simulink model "impulsestepmodel"  (Simulink 8.3)
settings: Solver=ode23tb  StartTime=0.0  StopTime=100  RelTol=1e-3
settings Model: Creator=NILIMESH GHOSH  LastModifiedBy=NILIMESH GHOSH
settings DataIOCC: SignalLoggingSaveFormat=Dataset
settings DebuggingCC: UnderspecifiedInitializationDetection=Simplified  SolverPrmCheckMsg=none  StateNameClashWarn=none
settings GRTTargetCC: CombineOutputUpdateFcns=on  GRTInterface=off

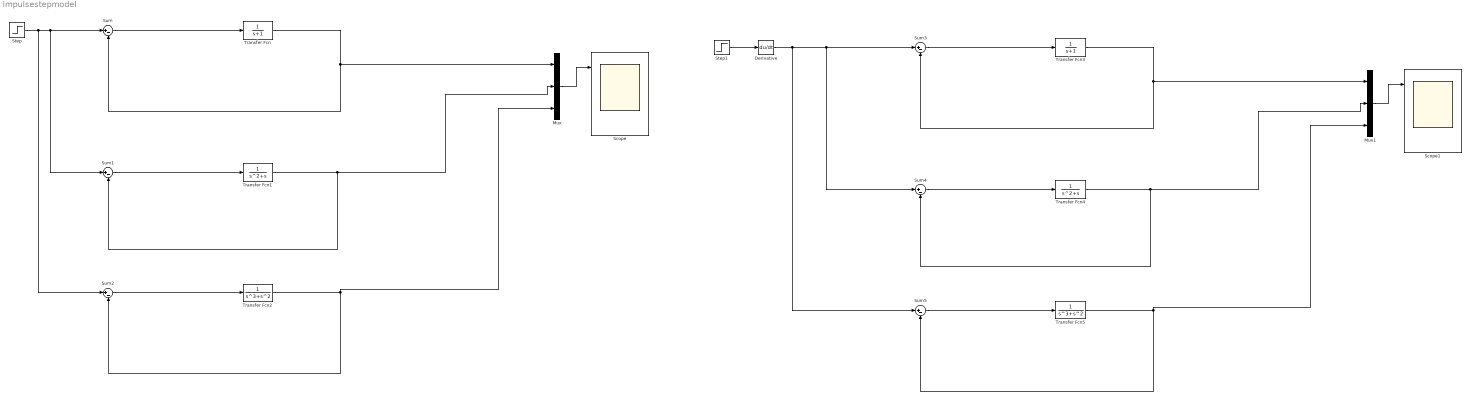
== system impulsestepmodel ==
  Derivative : Derivative
  Mux : Mux  Inputs=3
  Mux1 : Mux  Inputs=3
  Scope : Scope  NumInputPorts=3
      settings: TimeRange=100  YMin=-2~-5~-5  YMax=10~15~5
  Scope1 : Scope  NumInputPorts=3
      settings: TimeRange=100  YMin=-15000000000~-1~-1  YMax=35000000000~1~1
  Step : Step  Time=0  After=10  SampleTime=0  VectorParams1D=off  ZeroCross=off
  Step1 : Step  Time=0.01  After=10  SampleTime=0  VectorParams1D=off  ZeroCross=off
  Sum{,1..5} (6 alike) : Sum  Inputs=|+-
  Transfer Fcn : TransferFcn  Numerator=1  Denominator=[1 1]
  Transfer Fcn1 : TransferFcn  Numerator=1  Denominator=[1 1 0]
  Transfer Fcn2 : TransferFcn  Numerator=1  Denominator=[1 1 0 0]
  Transfer Fcn3 : TransferFcn  Numerator=1  Denominator=[1 1]
  Transfer Fcn4 : TransferFcn  Numerator=1  Denominator=[1 1 0]
  Transfer Fcn5 : TransferFcn  Numerator=1  Denominator=[1 1 0 0]
  wires:
  Sum/1 -> Transfer Fcn/1
  Transfer Fcn/1 -> Sum/2, Mux/1
  Sum1/1 -> Transfer Fcn1/1
  Transfer Fcn1/1 -> Mux/2, Sum1/2
  Sum2/1 -> Transfer Fcn2/1
  Step/1 -> Sum2/1, Sum1/1, Sum/1
  Transfer Fcn2/1 -> Mux/3, Sum2/2
  Mux/1 -> Scope/1
  Sum3/1 -> Transfer Fcn3/1
  Transfer Fcn3/1 -> Sum3/2, Mux1/1
  Sum4/1 -> Transfer Fcn4/1
  Transfer Fcn4/1 -> Mux1/2, Sum4/2
  Sum5/1 -> Transfer Fcn5/1
  Transfer Fcn5/1 -> Mux1/3, Sum5/2
  Mux1/1 -> Scope1/1
  Step1/1 -> Derivative/1
  Derivative/1 -> Sum5/1, Sum4/1, Sum3/1
